simulink model "mdlForRotoTransMatrices"  (R2014b)
settings: Solver=ode45  StartTime=0.0  StopTime=Ts  RelTol=1e-3
InitFcn:
  | setenv('YARP_ROBOT_NAME', 'icubGazeboSim');
  | ROBOT_DOF=25;
  | robotName='icubGazeboSim';
  | localName='simulink';
  | Ts=0.10;
libraries: WBCLibrary x2
settings Model: Creator=jorhabib  LastModifiedBy=jorhabib

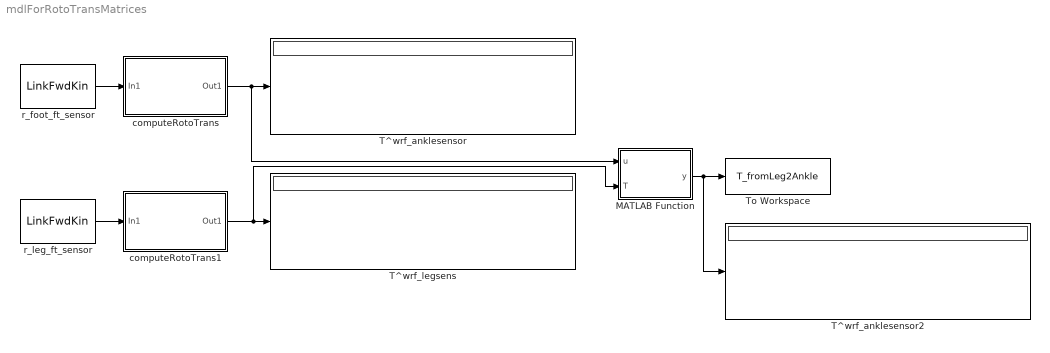
== system mdlForRotoTransMatrices ==
  MATLAB Function : MATLAB Function  TreatAsAtomicUnit=on
  T^wrf_anklesensor : Display
  T^wrf_anklesensor2 : Display
  T^wrf_legsens : Display
  To Workspace : ToWorkspace  VariableName=T_fromLeg2Ankle  SaveFormat=Timeseries  SampleTime=-1
  computeRotoTrans : Subsystem
  computeRotoTrans1 : Subsystem
  r_foot_ft_sensor : WBCLibrary/wholeBodyModel/Forward Kinematics/LinkFwdKin  robotname=robotName  localname=localName  link=r_foot
  r_leg_ft_sensor : WBCLibrary/wholeBodyModel/Forward Kinematics/LinkFwdKin  robotname=robotName  localname=localName  link=r_hip_3
  wires:
  r_foot_ft_sensor/1 -> computeRotoTrans/1(In1)
  computeRotoTrans/1(Out1) -> MATLAB Function/1(u), T^wrf_anklesensor/1
  r_leg_ft_sensor/1 -> computeRotoTrans1/1(In1)
  computeRotoTrans1/1(Out1) -> MATLAB Function/2(T), T^wrf_legsens/1
  MATLAB Function/1(y) -> T^wrf_anklesensor2/1, To Workspace/1

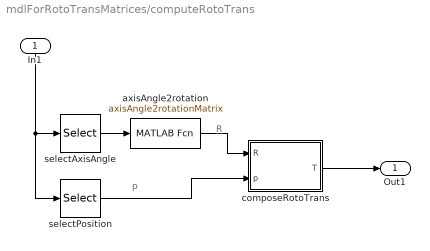
== system mdlForRotoTransMatrices/computeRotoTrans ==
  note: p
  note: R
  In1 : Inport
  axisAngle2rotation : MATLABFcn  MATLABFcn=axisAngle2rotationMatrix
  composeRotoTrans : MATLAB Function  TreatAsAtomicUnit=on
  selectAxisAngle : Selector  InputPortWidth=7  Indices=[4:7]
  selectPosition : Selector  InputPortWidth=7  Indices=[1:3]
  Out1 : Outport
  wires:
  axisAngle2rotation/1 -> composeRotoTrans/1(R)
  selectPosition/1 -> composeRotoTrans/2(p)
  In1/1 -> selectPosition/1, selectAxisAngle/1
  selectAxisAngle/1 -> axisAngle2rotation/1
  composeRotoTrans/1(T) -> Out1/1

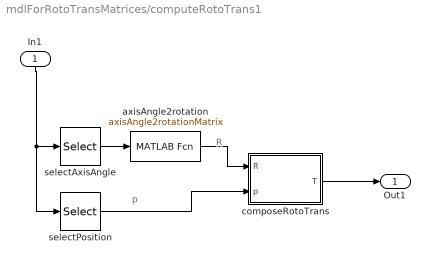
== system mdlForRotoTransMatrices/computeRotoTrans1 ==
  note: R
  note: p
  In1 : Inport
  axisAngle2rotation : MATLABFcn  MATLABFcn=axisAngle2rotationMatrix
  composeRotoTrans : MATLAB Function  TreatAsAtomicUnit=on
  selectAxisAngle : Selector  InputPortWidth=7  Indices=[4:7]
  selectPosition : Selector  InputPortWidth=7  Indices=[1:3]
  Out1 : Outport
  wires:
  composeRotoTrans/1(T) -> Out1/1
  selectAxisAngle/1 -> axisAngle2rotation/1
  In1/1 -> selectAxisAngle/1, selectPosition/1
  selectPosition/1 -> composeRotoTrans/2(p)
  axisAngle2rotation/1 -> composeRotoTrans/1(R)

== matlab function mdlForRotoTransMatrices/computeRotoTrans1/composeRotoTrans ==
  data: R input; T output; p input
function T = fcn(R, p)
%#codegen
R = reshape(R,3,3);

T = zeros(4,4);
T(end,:) = [0 0 0 1];
T(1:3, 1:3) = R;
T(1:3,end) = p;

== matlab function mdlForRotoTransMatrices/computeRotoTrans/composeRotoTrans ==
  data: R input; T output; p input
function T = fcn(R, p)
%#codegen
R = reshape(R,3,3);

T = zeros(4,4);
T(end,:) = [0 0 0 1];
T(1:3, 1:3) = R;
T(1:3,end) = p;

== matlab function mdlForRotoTransMatrices/MATLAB Function ==
  data: u input; y output; T input
function y = fcn(u, T)
%#codegen

y = u\T;
